simulink model "SimulatorUnityConnection"  (R2022b)
settings: configuration reference "WheelSimConfiguration" (kept outside this file)
undefined symbols (not defined in the file): simulator
settings Model: SimulationMode=external  Creator=MOSA  LastModifiedBy=MOSA
settings ConfigSetRef: SourceName=WheelSimConfiguration  SourceLocation=Base Workspace

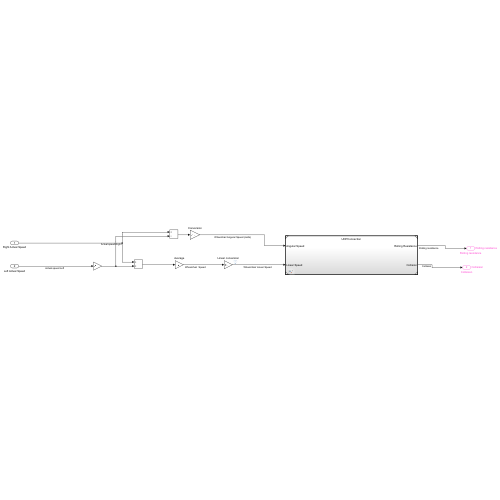
[thumbnail: Simulink's stored preview of the top-level diagram]
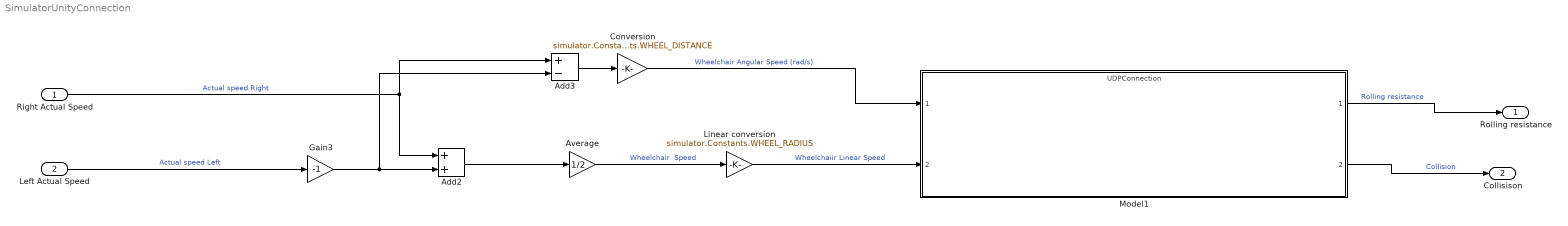
== system SimulatorUnityConnection ==
  Right Actual Speed : Inport
  Left Actual Speed : Inport  Port=2
  Add2 : Sum
  Add3 : Sum  Inputs=+-
  Average : Gain  Gain=1/2
  Conversion : Gain  Gain=simulator.Constants.WHEEL_RADIUS/simulator.Constants.WHEEL_DISTANCE
  Gain3 : Gain  Gain=-1
  Linear conversion : Gain  Gain=simulator.Constants.WHEEL_RADIUS
  Model1 : ModelReference  ModelNameDialog=UDPConnection.slx  SimulationMode=Normal  ModelReferenceVersion=1.71
  Rolling resistance : Outport  SignalName=Rolling resistance
  Collisison : Outport  Port=2  SignalName=Collisison
  wires:
  Add2/1 -> Average/1
  Add3/1 -> Conversion/1
  Model1/1 -> Rolling resistance/1  "Rolling resistance"
  Model1/2 -> Collisison/1  "Collision"
  Gain3/1 -> Add3/2, Add2/2
  Right Actual Speed/1 -> Add3/1, Add2/1  "Actual speed Right"
  Left Actual Speed/1 -> Gain3/1  "Actual speed Left"
  Linear conversion/1 -> Model1/2  "Wheelchaiir Linear Speed"
  Average/1 -> Linear conversion/1  "Wheelchair  Speed"
  Conversion/1 -> Model1/1  "Wheelchair Angular Speed (rad/s)"
